simulink subsystem "ControlerBA"  (R2023b)
settings: Solver=VariableStepAuto  StartTime=0.0  StopTime=10.0  RelTol=1e-3
settings Model: Creator=Usuario_UMA  LastModifiedBy=Manuel

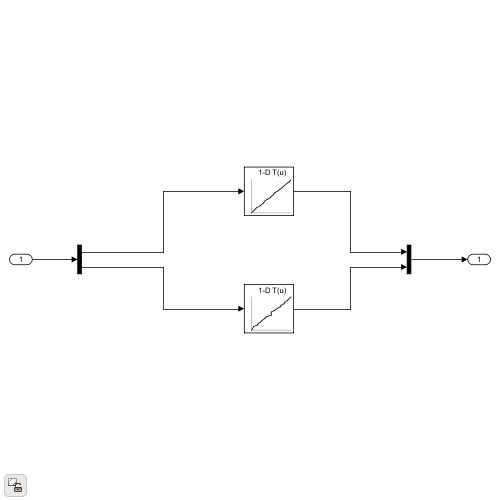
[thumbnail: Simulink's stored preview of the top-level diagram]
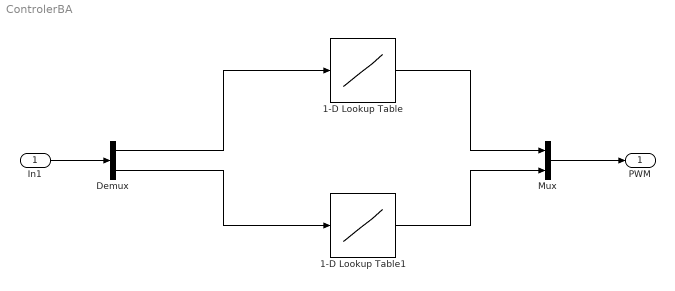
== system ControlerBA ==
  In1 : Inport
  1-D Lookup Table : Lookup_n-D  NumberOfTableDimensions=1  BreakpointsForDimension1=[-0.547622680664063;-0.435302734375;-0.393173217773438;-0.322952270507813;-0.280838012695313;-0.210617065429688;-0.168487548828125;-0.112350463867188;-0.007;0;0.070220947265625;0.112334728240967;0.196578979492188;0.238712310791016;0.308929443359375;0.351047515869141;0.477432250976563;0.519561767578125;0.547622680664063]  Table=[-254;-200.554992675781;-175.10498046875;-150.503311157227;-125.053283691406;-100.451629638672;-75.0016098022461;-50.3999557495117;-24.9500198364258;0;25.1016693115234;50.489990234375;75.1533508300781;100.470001220703;125.205039978027;150.449996948242;199.858367919922;220.218338012695;255]  InternalRulePriority=Speed  RndMeth=Simplest
  1-D Lookup Table1 : Lookup_n-D  NumberOfTableDimensions=1  BreakpointsForDimension1=[-0.519546508789063;-0.449333190917969;-0.365097045898438;-0.337005615234375;-0.266799926757813;-0.238710403442383;-0.15447998046875;-0.112334728240967;-7e-07;0;7e-08;0.126358032226563;0.168501853942871;0.238693237304688;0.266794204711914;0.351043701171875;0.365081787109375;0.4493408203125;0.491455078125;0.51953125]  Table=[-254;-200.15202331543;-175.10498046875;-150.876007080078;-125.053283691406;-100.076057434082;-75.0016098022461;-50.2919883728027;-24.9500198364258;0;24.9899826049805;50.5516815185547;74.9700088500977;100.603355407715;124.949989318848;149.806671142578;174.929992675781;199.858367919922;225.308334350586;255]  InternalRulePriority=Speed  RndMeth=Simplest
  Demux : Demux  Outputs=2
  Mux : Mux  Inputs=2
  PWM : Outport
  wires:
  Mux/1 -> PWM/1
  In1/1 -> Demux/1
  1-D Lookup Table1/1 -> Mux/2
  Demux/2 -> 1-D Lookup Table1/1
  Demux/1 -> 1-D Lookup Table/1
  1-D Lookup Table/1 -> Mux/1
